simulink library "tpm"  (R2021b)
settings: Solver=VariableStepAuto  StartTime=0.0  StopTime=10.0  RelTol=1e-3
undefined symbols (not defined in the file or in its folder): ENUM_AN_LF, ENUM_AN_LR, ENUM_AN_RF, ENUM_AN_RR, ENUM_POWERSTA_OFF, ENUM_POWERSTA_OFFA, ENUM_POWERSTA_OFFC, ENUM_POWERSTA_ON, ENUM_POWERSTA_READY, ENUM_POWERSTA_STANDBY, ENUM_PWRSTASW_OFF, ENUM_PWRSTASW_OFFA, ENUM_PWRSTASW_OFFCHVCHRG, ENUM_PWRSTASW_STANDBY, ENUM_TPMSSNESORIDREGSTA_START, FALSE, KTPM_DataInVehSpdThreshold_kph, KTPM_Delay_raw8, KTPM_DiagLearn_flg, KTPM_TPMSModelVersion_raw, KTPM_TPMSModelVersionInit_raw, KTPM_WhlRotDir_enum_ovrdflg, KTPM_WhlRotDir_enum_ovrdval, TRUE, ZERO_FLOAT, ZERO_INT
libraries: simulink x58, $bdroot x27, hcu_lib x24
(part 2 of 9)

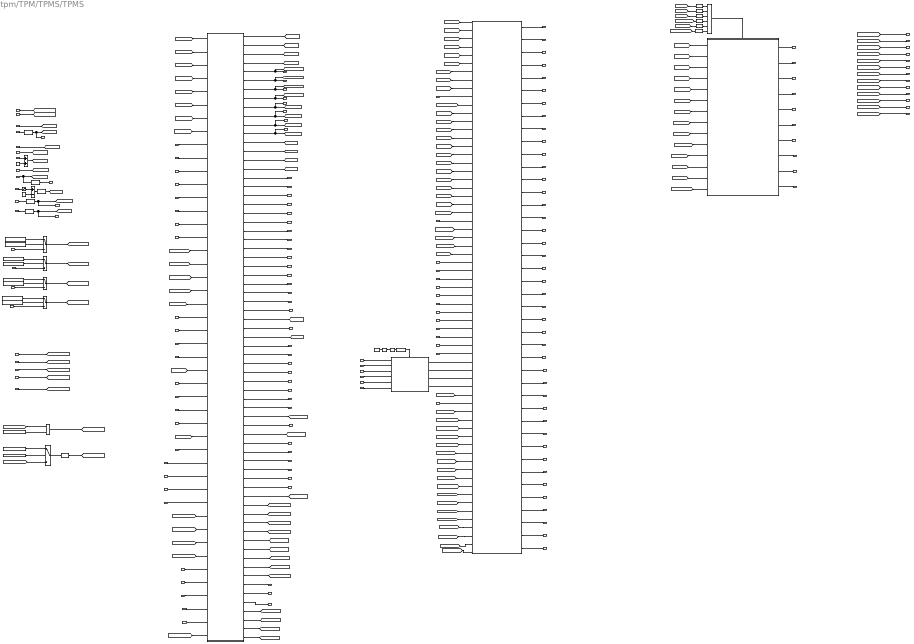
== system tpm/TPM/TPMS/TPMS ==
  note: VINP_RFWhlRotDir_enum
  VPMM_PowerSta_enum : Inport
  VINP_IDin_raw32 : Inport  Port=2
  VINP_DATAin_flg : Inport  Port=3
  VINP_FAT_flg : Inport  Port=4
  VINP_Pin_raw8 : Inport  Port=5
  VINP_Tin_raw8 : Inport  Port=6
  VINP_LFPulseCount_cnt : Inport  Port=7
  VINP_RFPulseCount_cnt : Inport  Port=8
  VINP_LRPulseCount_cnt : Inport  Port=9
  VINP_RRPulseCount_cnt : Inport  Port=10
  VINP_LFPulseCountV_flg : Inport  Port=11
  VINP_RFPulseCountV_flg : Inport  Port=12
  VINP_LRPulseCountV_flg : Inport  Port=13
  VINP_RRPulseCountV_flg : Inport  Port=14
  VINP_BatteryLow_flg : Inport  Port=15
  VTQD_GearActualPosn_enum : Inport  Port=16
  VINP_VehSpeed_kph : Inport  Port=17
  VINP_TPMSResButt_flg : Inport  Port=18
  VINP_TPMSCaliButt_flg : Inport  Port=19
  VINP_IVICANValid_flg : Inport  Port=20
  VINP_TPMSStorge_flg : Inport  Port=21
  VINP_LFID_raw : Inport  Port=22
  VINP_RFID_raw : Inport  Port=23
  VINP_LRID_raw : Inport  Port=24
  VINP_RRID_raw : Inport  Port=25
  VINP_ChkStorge_flg : Inport  Port=26
  VINP_ChkLFID_raw : Inport  Port=27
  VINP_ChkRFID_raw : Inport  Port=28
  VINP_ChkLRID_raw : Inport  Port=29
  VINP_ChkRRID_raw : Inport  Port=30
  VINP_LFWhlRotDir_enum : Inport  Port=31
  VINP_RFWhlRotDir_enum : Inport  Port=32
  VINP_LRWhlRotDir_enum : Inport  Port=33
  VINP_RRWhlRotDir_enum : Inport  Port=34
  VINP_FlashLFSensorFail_flg : Inport  Port=35
  VINP_FlashRFSensorFail_flg : Inport  Port=36
  VINP_FlashLRSensorFail_flg : Inport  Port=37
  VINP_FlashRRSensorFail_flg : Inport  Port=38
  VINP_FlashLFWheelPSW_raw8 : Inport  Port=39
  VINP_FlashRFWheelPSW_raw8 : Inport  Port=40
  VINP_FlashLRWheelPSW_raw8 : Inport  Port=41
  VINP_FlashRRWheelPSW_raw8 : Inport  Port=42
  VINP_FlashLFPindi_enum : Inport  Port=43
  VINP_FlashRFPindi_enum : Inport  Port=44
  VINP_FlashLRPindi_enum : Inport  Port=45
  VINP_FlashRRPindi_enum : Inport  Port=46
  VINP_FlashLFP20_raw8 : Inport  Port=47
  VINP_FlashRFP20_raw8 : Inport  Port=48
  VINP_FlashLRP20_raw8 : Inport  Port=49
  VINP_FlashRRP20_raw8 : Inport  Port=50
  VINP_FlashLFWheelPress_raw8 : Inport  Port=51
  VINP_FlashRFWheelPress_raw8 : Inport  Port=52
  VINP_FlashLRFWheelPress_raw8 : Inport  Port=53
  VINP_FlashRRWheelPress_raw8 : Inport  Port=54
  VINP_FlashLFWheelTemp_C : Inport  Port=55
  VINP_FlashRFWheelTemp_C : Inport  Port=56
  VINP_FlashLRWheelTemp_C : Inport  Port=57
  VINP_FlashRRWheelTemp_C : Inport  Port=58
  VINP_FlashunlearnSfali_flg : Inport  Port=59
  VINP_S1ID_raw : Inport  Port=60
  VINP_S2ID_raw : Inport  Port=61
  VINP_S3ID_raw : Inport  Port=62
  VINP_S4ID_raw : Inport  Port=63
  VINP_Prepresstemptrust_flg : Inport  Port=64
  VINP_TPMSTrigger_flg : Inport  Port=65
  VINP_TPMSSensorIDRegSta_enum : Inport  Port=66
  VINP_FlashTPMModelVersion_raw : Inport  Port=67
  VINP_FlashTPMModelVersionChkSum_raw : Inport  Port=68
  Add : Sum  OutDataTypeStr=int8
  Add1 : Sum  Inputs=+-
  Cast To Boolean : DataTypeConversion  OutDataTypeStr=boolean
  Constant : Constant  Value=-40
  Constant1 : Constant  Value=59
  Constant{5,7,10..11} (4 alike) : Constant  Value=KTPM_WhlRotDir_enum_ovrdflg
  Constant12 : Constant  Value=ENUM_TPMSSNESORIDREGSTA_START
  Constant13 : Constant  Value=TRUE
  Constant{2..4,6} (4 alike) : Constant  Value=KTPM_WhlRotDir_enum_ovrdval
  Constant8 : Constant  Value=KTPM_DiagLearn_flg
  Constant9 : Constant  Value=TRUE
  Data Type Conversion : DataTypeConversion  OutDataTypeStr=uint8
  Data Type Conversion1 : DataTypeConversion  OutDataTypeStr=uint32
  Data Type Conversion2 : DataTypeConversion  OutDataTypeStr=boolean
  Data Type Conversion3 : DataTypeConversion  OutDataTypeStr=boolean
  Data Type Conversion4 : DataTypeConversion  OutDataTypeStr=boolean
  Delay : Delay
  Detect Increase{,1..6} (7 alike) : simulink/Logic and Bit Operations/Detect Increase  vinit=0.0  OutDataTypeStr=boolean
  Equal : RelationalOperator  Operator===  OutDataTypeStr=boolean  RndMeth=Simplest
  GetFlashWheelTemp : Subsystem
  Learn : Subsystem
  Logical Operator : Logic  Operator=OR  Inputs=6  AllPortsSameDT=off  OutDataTypeStr=boolean
  Logical Operator1 : Logic  Operator=NOT  AllPortsSameDT=off  OutDataTypeStr=boolean
  Saturation : Saturate  UpperLimit=255  LowerLimit=59
  Send : Subsystem
  Subsystem : Subsystem
  Switch : Switch  Criteria=u2 > Threshold
  Switch{2..5} (4 alike) : Switch  Criteria=u2 ~= 0
  "VTPM_LFBatWarn_flg " : Outport
  "VTPM_RFBatWarn_flg " : Outport  Port=2
  "VTPM_LRBatWarn_flg " : Outport  Port=3
  "VTPM_RRBatWarn_flg " : Outport  Port=4
  VTPM_LFWheelPress_raw8 : Outport  Port=5
  VTPM_RFWheelPress_raw8 : Outport  Port=6
  VTPM_LRWheelPress_raw8 : Outport  Port=7
  VTPM_RRWheelPress_raw8 : Outport  Port=8
  "VTPM_LFWheelTemp_C " : Outport  Port=9
  "VTPM_RFWheelTemp_C " : Outport  Port=10
  "VTPM_LRWheelTemp_C " : Outport  Port=11
  VTPM_RRWheelTemp_C : Outport  Port=12
  VTPM_LFSensorFail_flg : Outport  Port=13
  VTPM_RFSensorFail_flg : Outport  Port=14
  VTPM_LRSensorFail_flg : Outport  Port=15
  VTPM_RRSensorFail_flg : Outport  Port=16
  VTPM_LFWheelDebug_flg : Outport  Port=17
  VTPM_LRWheelDebug_flg : Outport  Port=18
  VTPM_RFWheelDebug_flg : Outport  Port=19
  VTPM_RRWheelDebug_flg : Outport  Port=20
  VTPM_TPMSResButtAllow_flg : Outport  Port=21
  VTPM_TPMSCaliButtAllow_flg : Outport  Port=22
  VTPM_LFPressIndi_enum : Outport  Port=23
  VTPM_RFPressIndi_enum : Outport  Port=24
  VTPM_LRPressIndi_enum : Outport  Port=25
  VTPM_RRPressIndi_enum : Outport  Port=26
  "VTPM_TPMSWarnIndi_enum " : Outport  Port=27
  VTPM_LFWheelTmpIndi_flg : Outport  Port=28
  VTPM_RFWheelTmpIndi_flg : Outport  Port=29
  VTPM_LRWheelTmpIndi_flg : Outport  Port=30
  VTPM_RRWheelTmpIndi_flg : Outport  Port=31
  VTPM_LFWheelPSW_raw8 : Outport  Port=32
  VTPM_LRWheelPSW_raw8 : Outport  Port=33
  VTPM_RFWheelPSW_raw8 : Outport  Port=34
  VTPM_RRWheelPSW_raw8 : Outport  Port=35
  VTPM_CWheelTips_enum : Outport  Port=36
  VTPM_AutoLTips_enum : Outport  Port=37
  VTPM_LFSensorMode_flg : Outport  Port=38
  VTPM_RFSensorMode_flg : Outport  Port=39
  VTPM_LRSensorMode_flg : Outport  Port=40
  VTPM_RRSensorMode_flg : Outport  Port=41
  VTPM_LFS1_cnt : Outport  Port=42
  VTPM_RFS1_cnt : Outport  Port=43
  VTPM_RRS1_cnt : Outport  Port=44
  VTPM_LRS1_cnt : Outport  Port=45
  VTPM_LFS2_cnt : Outport  Port=46
  VTPM_RFS2_cnt : Outport  Port=47
  VTPM_RRS2_cnt : Outport  Port=48
  VTPM_LRS2_cnt : Outport  Port=49
  VTPM_LFS3_cnt : Outport  Port=50
  VTPM_RFS3_cnt : Outport  Port=51
  VTPM_RRS3_cnt : Outport  Port=52
  VTPM_LRS3_cnt : Outport  Port=53
  VTPM_LFS4_cnt : Outport  Port=54
  VTPM_RFS4_cnt : Outport  Port=55
  VTPM_RRS4_cnt : Outport  Port=56
  VTPM_LRS4_cnt : Outport  Port=57
  VTPM_S1ID_raw32 : Outport  Port=58
  VTPM_S2ID_raw32 : Outport  Port=59
  VTPM_S3ID_raw32 : Outport  Port=60
  VTPM_S4ID_raw32 : Outport  Port=61
  VTPM_S1L_enum : Outport  Port=62
  VTPM_S2L_enum : Outport  Port=63
  VTPM_S3L_enum : Outport  Port=64
  VTPM_S4L_enum : Outport  Port=65
  VTPM_ALFin_flg : Outport  Port=66
  VTPM_IDLOCK_flg : Outport  Port=67
  VTPM_LFP20_raw8 : Outport  Port=68
  VTPM_RFP20_raw8 : Outport  Port=69
  VTPM_LRP20_raw8 : Outport  Port=70
  VTPM_RRP20_raw8 : Outport  Port=71
  VTPM_FAT_flg : Outport  Port=72
  VTPM_IDin_raw32 : Outport  Port=73
  VTPM_S1WheelDebugALTU_pct : Outport  Port=74
  VTPM_S2WheelDebugALTU_pct : Outport  Port=75
  VTPM_S3WheelDebugALTU_pct : Outport  Port=76
  VTPM_S4WheelDebugALTU_pct : Outport  Port=77
  VTPM_ID1messageALTU_raw8 : Outport  Port=78
  VTPM_ID2messageALTU_raw8 : Outport  Port=79
  VTPM_ID3messageALTU_raw8 : Outport  Port=80
  VTPM_ID4messageALTU_raw8 : Outport  Port=81
  VTPM_Chkfin_flg : Outport  Port=82
  VTPM_SetIDLoc_flg : Outport  Port=83
  VTPM_TPMSStorge_flg : Outport  Port=84
  VTPM_ChkStorge_flg : Outport  Port=85
  VTPM_TPMSResButt_flg : Outport  Port=86
  VTPM_LFPindi_enum : Outport  Port=87
  VTPM_RFPind_enum : Outport  Port=88
  VTPM_LRPindi_enum : Outport  Port=89
  VTPM_RRPindi_enum : Outport  Port=90
  VTPM_WriteChkLFID_raw : Outport  Port=91
  VTPM_WriteChkRFID_raw : Outport  Port=92
  VTPM_WriteChkLRID_raw : Outport  Port=93
  VTPM_WriteChkRRID_raw : Outport  Port=94
  VTPM_WriteChkfinLFID_raw : Outport  Port=95
  VTPM_WriteChkfinRFID_raw : Outport  Port=96
  VTPM_WriteChkfinLRID_raw : Outport  Port=97
  VTPM_WriteChkfinRRID_raw : Outport  Port=98
  VTPM_Flashchkdatavalid_enum : Outport  Port=99
  VTPM_Flashdatavalid_enum : Outport  Port=100
  VTPM_unlearnSfali_flg : Outport  Port=101
  VTPM_unlearnSfailvalid_enum : Outport  Port=102
  VTPM_Prepresstempvalid_enum : Outport  Port=103
  VTPM_FlashS1ID_raw : Outport  Port=104
  VTPM_FlashS2ID_raw : Outport  Port=105
  VTPM_FlashS3ID_raw : Outport  Port=106
  VTPM_FlashS4ID_raw : Outport  Port=107
  VTPM_FlashIDvalid_enum : Outport  Port=108
  VTPM_WritingCnt_enum : Outport  Port=109
  VTPM_TPMSTLCmd_flg : Outport  Port=110
  VTPM_LProgress_enum : Outport  Port=111
  VTPM_TPMSSensorIDRegStart_flg : Outport  Port=112
  wires:
  Add/1 -> [VINP_Tin_raw8]
  VINP_Tin_raw8/1 -> Add/1
  Constant/1 -> Add/2
  VINP_TPMSCaliButt_flg/1 -> [VINP_TPMSCaliButt_flg]
  VINP_TPMSResButt_flg/1 -> Data Type Conversion4/1
  VINP_IDin_raw32/1 -> Data Type Conversion1/1, [VINP_IDin_raw32]
  VPMM_PowerSta_enum/1 -> [VPMM_PowerSta_enum]
  Constant1/1 -> Add1/2
  VINP_Pin_raw8/1 -> Saturation/1
  Data Type Conversion/1 -> [VINP_Pin_raw8]
  Saturation/1 -> Add1/1
  Add1/1 -> Data Type Conversion/1
  Data Type Conversion1/1 -> VTPM_IDin_raw32/1
  VINP_VehSpeed_kph/1 -> [VINP_VehSpeed_kph]
  Constant10/1 -> Switch4/2
  Constant7/1 -> Switch3/2
  VINP_LRWhlRotDir_enum/1 -> Switch4/3
  Constant3/1 -> Switch2/1
  Constant5/1 -> Switch2/2
  Constant4/1 -> Switch4/1
  VINP_RFWhlRotDir_enum/1 -> Switch2/3
  Constant2/1 -> Switch3/1
  VINP_LFWhlRotDir_enum/1 -> Switch3/3
  VINP_RRWhlRotDir_enum/1 -> Switch5/3
  Constant11/1 -> Switch5/2
  Constant6/1 -> Switch5/1
  Switch5/1 -> [VTPM_RRWhlRotDir_enum]
  Switch4/1 -> [VTPM_LRWhlRotDir_enum]
  Switch2/1 -> [VTPM_RFWhlRotDir_enum]
  Switch3/1 -> [VTPM_LFWhlRotDir_enum]
  [VTPM_LRWhlRotDir_enum] -> Learn/19(VTPM_LRWhlRotDir_enum)
  [VTPM_RRWhlRotDir_enum] -> Learn/20(VTPM_RRWhlRotDir_enum)
  [VTPM_LFWhlRotDir_enum] -> Learn/17(VTPM_LFWhlRotDir_enum)
  [VTPM_RFWhlRotDir_enum] -> Learn/18(VTPM_RFWhlRotDir_enum)
  [VINP_TPMSStorge_flg] -> Learn/21(VINP_TPMSStorge_flg)
  VINP_LFID_raw/1 -> Learn/22(VINP_LFID_raw)
  VINP_RFID_raw/1 -> Learn/23(VINP_RFID_raw)
  VINP_LRID_raw/1 -> Learn/24(VINP_LRID_raw)
  VINP_RRID_raw/1 -> Learn/25(VINP_RRID_raw)
  VINP_ChkLFID_raw/1 -> Learn/27(VINP_ChkLFID_raw)
  VINP_ChkRFID_raw/1 -> Learn/28(VINP_ChkRFID_raw)
  VINP_ChkLRID_raw/1 -> Learn/29(VINP_ChkLRID_raw)
  VINP_ChkRRID_raw/1 -> Learn/30(VINP_ChkRRID_raw)
  Learn/43(VTPM_ID4messageALTU_raw8) -> VTPM_ID4messageALTU_raw8/1
  Learn/5(VTPM_LFWheelPSW_raw8) -> [VTPM_LFWheelPSW_raw8], VTPM_LFWheelPSW_raw8/1
  Learn/6(VTPM_RFWheelPSW_raw8) -> [VTPM_RFWheelPSW_raw8], VTPM_RFWheelPSW_raw8/1
  Learn/7(VTPM_LRWheelPSW_raw8) -> [VTPM_LRWheelPSW_raw8], VTPM_LRWheelPSW_raw8/1
  Learn/8(VTPM_RRWheelPSW_raw8) -> [VTPM_RRWheelPSW_raw8], VTPM_RRWheelPSW_raw8/1
  Learn/9(VTPM_LFLowPind_enum) -> VTPM_LFPindi_enum/1, [VTPM_LFLowPind_enum]
  Learn/10(VTPM_RFLowPind_enum) -> VTPM_RFPind_enum/1, [VTPM_RFLowPind_enum]
  Learn/11(VTPM_LRLowPind_enum) -> VTPM_LRPindi_enum/1, [VTPM_LRLowPind_enum]
  Learn/12(VTPM_RRLowPind_enum) -> VTPM_RRPindi_enum/1, [VTPM_RRLowPind_enum]
  Learn/1(VTPM_S1ID_raw32) -> [VTPM_S1ID_raw32]
  Learn/2(VTPM_S2ID_raw32) -> [VTPM_S2ID_raw32]
  Learn/3(VTPM_S3ID_raw32) -> [VTPM_S3ID_raw32]
  Learn/4(VTPM_S4ID_raw32) -> [VTPM_S4ID_raw32]
  Learn/17(VTPM_LFS1_cnt) -> VTPM_LFS1_cnt/1
  Learn/18(VTPM_RFS1_cnt) -> VTPM_RFS1_cnt/1
  Learn/19(VTPM_RRS1_cnt) -> VTPM_RRS1_cnt/1
  Learn/20(VTPM_LRS1_cnt) -> VTPM_LRS1_cnt/1
  Learn/21(VTPM_LFS2_cnt) -> VTPM_LFS2_cnt/1
  Learn/22(VTPM_RFS2_cnt) -> VTPM_RFS2_cnt/1
  Learn/23(VTPM_RRS2_cnt) -> VTPM_RRS2_cnt/1
  Learn/24(VTPM_LRS2_cnt) -> VTPM_LRS2_cnt/1
  Learn/25(VTPM_LFS3_cnt) -> VTPM_LFS3_cnt/1
  Learn/26(VTPM_RFS3_cnt) -> VTPM_RFS3_cnt/1
  Learn/27(VTPM_RRS3_cnt) -> VTPM_RRS3_cnt/1
  Learn/28(VTPM_LRS3_cnt) -> VTPM_LRS3_cnt/1
  Learn/29(VTPM_LFS4_cnt) -> VTPM_LFS4_cnt/1
  Learn/30(VTPM_RFS4_cnt) -> VTPM_RFS4_cnt/1
  Learn/31(VTPM_RRS4_cnt) -> VTPM_RRS4_cnt/1
  Learn/32(VTPM_LRS4_cnt) -> VTPM_LRS4_cnt/1
  Learn/39(VTPM_S4WheelDebugALTU_pct) -> VTPM_S4WheelDebugALTU_pct/1
  Learn/40(VTPM_ID1messageALTU_raw8) -> VTPM_ID1messageALTU_raw8/1
  Learn/41(VTPM_ID2messageALTU_raw8) -> VTPM_ID2messageALTU_raw8/1
  Learn/42(VTPM_ID3messageALTU_raw8) -> VTPM_ID3messageALTU_raw8/1
  VTQD_GearActualPosn_enum/1 -> [VTQD_GearActualPosn_enum]
  [VINP_ChkStorge_flg] -> Learn/26(VINP_ChkStorge_flg)
  VINP_TPMSStorge_flg/1 -> Data Type Conversion2/1
  VINP_ChkStorge_flg/1 -> Data Type Conversion3/1
  [VTQD_GearActualPosn_enum] -> Send/11(VTQD_GearActualPosn_enum)
  [VTPM_ALFin_flg] -> Send/26(VTPM_ALFin_flg)
  [VINP_TPMSStorge_flg] -> Send/27(VINP_TPMSStorge_flg)
  [VTPM_IDLOCK_flg] -> Send/28(VTPM_IDLOCK_flg)
  [VINP_VehSpeed_kph] -> Send/12(VINP_VehSpeed_kph)
  [VINP_TPMSResButt_flg] -> Send/13(VINP_TPMSResButt_flg)
  [VINP_TPMSCaliButt_flg] -> Send/14(VINP_TPMSCaliButt_flg)
  [VTPM_S1L_enum] -> Send/15(VTPM_S1L_enum)
  [VTPM_S2L_enum] -> Send/16(VTPM_S2L_enum)
  [VTPM_S3L_enum] -> Send/17(VTPM_S3L_enum)
  [VTPM_S4L_enum] -> Send/18(VTPM_S4L_enum)
  [VTPM_Chkfin_flg] -> Send/19(VTPM_Chkfin_flg)
  [VTPM_LFLowPind_enum] -> Send/20(VTPM_LFLowPind_enum)
  [VTPM_RFLowPind_enum] -> Send/21(VTPM_RFLowPind_enum)
  [VTPM_LRLowPind_enum] -> Send/22(VTPM_LRLowPind_enum)
  [VTPM_RRLowPind_enum] -> Send/23(VTPM_RRLowPind_enum)
  [VINP_FAT_flg] -> Send/24(VINP_FAT_flg)
  [VPMM_PowerSta_enum] -> Send/1(VPMM_PowerSta_enum)
  [VTPM_S1ID_raw32] -> Send/2(VTPM_S1ID_raw32)
  [VTPM_S2ID_raw32] -> Send/3(VTPM_S2ID_raw32)
  [VTPM_S3ID_raw32] -> Send/4(VTPM_S3ID_raw32)
  [VTPM_S4ID_raw32] -> Send/5(VTPM_S4ID_raw32)
  [VINP_IDin_raw32] -> Send/6(VINP_IDin_raw32)
  [VINP_DATAin_flg] -> Send/7(VINP_DATAin_flg)
  [VINP_Pin_raw8] -> Send/8(VINP_Pin_raw8)
  [VINP_Tin_raw8] -> Send/9(VINP_Tin_raw8)
  [VINP_ChkStorge_flg] -> Send/29(VINP_ChkStorge_flg)
  VINP_IVICANValid_flg/1 -> Send/25(VINP_IVICANValid_flg)
  VINP_FlashLFSensorFail_flg/1 -> Send/30(VINP_FlashLFSensorFail_flg)
  VINP_FlashRFSensorFail_flg/1 -> Send/31(VINP_FlashRFSensorFail_flg)
  VINP_FlashLRSensorFail_flg/1 -> Send/32(VINP_FlashLRSensorFail_flg)
  VINP_FlashRRSensorFail_flg/1 -> Send/33(VINP_FlashRRSensorFail_flg)
  VINP_FlashLFP20_raw8/1 -> Send/34(VINP_FlashLFP20_raw8)
  VINP_FlashRFP20_raw8/1 -> Send/35(VINP_FlashRFP20_raw8)
  VINP_FlashLRP20_raw8/1 -> Send/36(VINP_FlashLRP20_raw8)
  VINP_FlashRRP20_raw8/1 -> Send/37(VINP_FlashRRP20_raw8)
  VINP_BatteryLow_flg/1 -> Send/10(VINP_BatteryLow_flg)
  VINP_FlashLFWheelPress_raw8/1 -> Send/38(VINP_FlashLFWheelPress_raw8)
  VINP_FlashRFWheelPress_raw8/1 -> Send/39(VINP_FlashRFWheelPress_raw8)
  VINP_FlashLRFWheelPress_raw8/1 -> Send/40(VINP_FlashLRFWheelPress_raw8)
  VINP_FlashRRWheelPress_raw8/1 -> Send/41(VINP_FlashRRWheelPress_raw8)
  [VTPM_S4L_enum] -> Subsystem/8(VTPM_S4L_enum)
  [VTPM_S3L_enum] -> Subsystem/7(VTPM_S3L_enum)
  [VTPM_S2L_enum] -> Subsystem/6(VTPM_S2L_enum)
  [VTPM_S2ID_raw32] -> Subsystem/2(VTPM_S2ID_raw32)
  [VTPM_S4ID_raw32] -> Subsystem/4(VTPM_S4ID_raw32)
  [VTPM_S3ID_raw32] -> Subsystem/3(VTPM_S3ID_raw32)
  [VINP_TPMSResButt_flg] -> Subsystem/13(VINP_TPMSResButt_flg)
  [VTPM_Chkfin_flg] -> Subsystem/10(VTPM_Chkfin_flg)
  [VTPM_S1L_enum] -> Subsystem/5(VTPM_S1L_enum)
  [VINP_TPMSStorge_flg] -> Subsystem/11(VINP_TPMSStorge_flg)
  [VINP_ChkStorge_flg] -> Subsystem/12(VINP_ChkStorge_flg)
  [VTPM_S1ID_raw32] -> Subsystem/1(VTPM_S1ID_raw32)
  [VTPM_ALFin_flg] -> Subsystem/9(VTPM_ALFin_flg)
  Logical Operator/1 -> Subsystem/Enable
  [VINP_TPMSStorge_flg] -> Detect Increase3/1
  Detect Increase3/1 -> Logical Operator/4
  [VTPM_ALFin_flg] -> Detect Increase/1
  [VINP_ChkStorge_flg] -> Detect Increase1/1
  [VTPM_Chkfin_flg] -> Detect Increase2/1
  Detect Increase/1 -> Logical Operator/1
  Detect Increase1/1 -> Logical Operator/2
  Detect Increase2/1 -> Logical Operator/3
  [VINP_TPMSResButt_flg] -> Detect Increase4/1
  Detect Increase4/1 -> Logical Operator/5
  Subsystem/1(VTPM_WriteChkLFID_raw) -> VTPM_WriteChkLFID_raw/1
  Subsystem/2(VTPM_WriteChkRFID_raw) -> VTPM_WriteChkRFID_raw/1
  Subsystem/3(VTPM_WriteChkLRID_raw) -> VTPM_WriteChkLRID_raw/1
  Subsystem/4(VTPM_WriteChkRRID_raw) -> VTPM_WriteChkRRID_raw/1
  Subsystem/5(VTPM_WriteChkfinLFID_raw) -> VTPM_WriteChkfinLFID_raw/1
  Subsystem/6(VTPM_WriteChkfinRFID_raw) -> VTPM_WriteChkfinRFID_raw/1
  Subsystem/7(VTPM_WriteChkfinLRID_raw) -> VTPM_WriteChkfinLRID_raw/1
  Subsystem/8(VTPM_WriteChkfinRRID_raw) -> VTPM_WriteChkfinRRID_raw/1
  Subsystem/9(VTPM_Flashchkdatavalid_enum) -> VTPM_Flashchkdatavalid_enum/1
  Subsystem/10(VTPM_Flashdatavalid_enum) -> VTPM_Flashdatavalid_enum/1
  [VTPM_unlearnSfali_flg] -> Send/46(VTPM_unlearnSfali_flg)
  [VINP_VehSpeed_kph] -> Learn/31(VINP_VehSpeed_kph)
  VINP_FlashunlearnSfali_flg/1 -> Learn/32(VINP_FlashunlearnSfali_flg)
  VINP_RRPulseCountV_flg/1 -> Learn/16(VINP_RRPulseCountV_flg)
  [VINP_TPMSResButt_flg] -> Learn/1(VINP_TPMSResButt_flg)
  [VINP_IDin_raw32] -> Learn/2(VINP_IDin_raw32)
  [VINP_DATAin_flg] -> Learn/3(VINP_DATAin_flg)
  [VINP_Pin_raw8] -> Learn/4(VINP_Pin_raw8)
  [VINP_Tin_raw8] -> Learn/5(VINP_Tin_raw8)
  [VINP_TPMSCaliButt_flg] -> Learn/6(VINP_TPMSCaliButt_flg)
  [VINP_FAT_flg] -> Learn/7(VINP_FAT_flg)
  [VPMM_PowerSta_enum] -> Learn/8(VPMM_PowerSta_enum)
  VINP_LFPulseCount_cnt/1 -> Learn/9(VINP_LFPulseCount_cnt)
  VINP_RFPulseCount_cnt/1 -> Learn/10(VINP_RFPulseCount_cnt)
  VINP_LRPulseCount_cnt/1 -> Learn/11(VINP_LRPulseCount_cnt)
  VINP_RRPulseCount_cnt/1 -> Learn/12(VINP_RRPulseCount_cnt)
  VINP_LFPulseCountV_flg/1 -> Learn/13(VINP_LFPulseCountV_flg)
  VINP_RFPulseCountV_flg/1 -> Learn/14(VINP_RFPulseCountV_flg)
  VINP_LRPulseCountV_flg/1 -> Learn/15(VINP_LRPulseCountV_flg)
  VINP_DATAin_flg/1 -> [VINP_DATAin_flg]
  VINP_FAT_flg/1 -> [VINP_FAT_flg]
  Data Type Conversion2/1 -> VTPM_TPMSStorge_flg/1, [VINP_TPMSStorge_flg]
  Data Type Conversion3/1 -> VTPM_ChkStorge_flg/1, [VINP_ChkStorge_flg]
  Data Type Conversion4/1 -> VTPM_TPMSResButt_flg/1, [VINP_TPMSResButt_flg]
  VINP_FlashLFPindi_enum/1 -> [VINP_FlashLFPindi_enum]
  VINP_FlashRFPindi_enum/1 -> [VINP_FlashRFPindi_enum]
  VINP_FlashLRPindi_enum/1 -> [VINP_FlashLRPindi_enum]
  VINP_FlashRRPindi_enum/1 -> [VINP_FlashRRPindi_enum]
  VINP_FlashLFWheelPSW_raw8/1 -> Learn/33(VINP_FlashLFWheelPSW_raw8)
  VINP_FlashRFWheelPSW_raw8/1 -> Learn/34(VINP_FlashRFWheelPSW_raw8)
  VINP_FlashLRWheelPSW_raw8/1 -> Learn/35(VINP_FlashLRWheelPSW_raw8)
  VINP_FlashRRWheelPSW_raw8/1 -> Learn/36(VINP_FlashRRWheelPSW_raw8)
  [VINP_FlashLFPindi_enum] -> Learn/37(VINP_FlashLFPindi_enum)
  [VINP_FlashRFPindi_enum] -> Learn/38(VINP_FlashRFPindi_enum)
  [VINP_FlashLRPindi_enum] -> Learn/39(VINP_FlashLRPindi_enum)
  [VINP_FlashRRPindi_enum] -> Learn/40(VINP_FlashRRPindi_enum)
  VINP_S3ID_raw/1 -> Learn/43(VINP_S3ID_raw)
  VINP_S4ID_raw/1 -> Learn/44(VINP_S4ID_raw)
  VINP_S2ID_raw/1 -> Learn/42(VINP_S2ID_raw)
  VINP_S1ID_raw/1 -> Learn/41(VINP_S1ID_raw)
  Learn/13(VTPM_S1L_enum) -> [VTPM_S1L_enum]
  Learn/16(VTPM_S4L_enum) -> [VTPM_S4L_enum]
  Learn/14(VTPM_S2L_enum) -> [VTPM_S2L_enum]
  Learn/15(VTPM_S3L_enum) -> [VTPM_S3L_enum]
  Learn/38(VTPM_S3WheelDebugALTU_pct) -> VTPM_S3WheelDebugALTU_pct/1
  Learn/33(VTPM_IDLOCK_flg) -> [VTPM_IDLOCK_flg]
  Learn/34(VTPM_FATAND_flg) -> VTPM_FAT_flg/1
  Learn/35(VTPM_ALFin_flg) -> [VTPM_ALFin_flg]
  Learn/36(VTPM_S1WheelDebugALTU_pct) -> VTPM_S1WheelDebugALTU_pct/1
  Learn/37(VTPM_S2WheelDebugALTU_pct) -> VTPM_S2WheelDebugALTU_pct/1
  Learn/44(VTPM_Chkfin_flg) -> [VTPM_Chkfin_flg]
  Learn/45(VTPM_SetIDLoc_flg) -> VTPM_SetIDLoc_flg/1
  Learn/46(VTPM_unlearnSfali_flg) -> [VTPM_unlearnSfali_flg]
  Learn/47(VTPM_unlearnSfailvalid_enum) -> VTPM_unlearnSfailvalid_enum/1
  Learn/48(VTPM_FlashS1ID_raw) -> VTPM_FlashS1ID_raw/1
  Learn/49(VTPM_FlashS2ID_raw) -> VTPM_FlashS2ID_raw/1
  Learn/50(VTPM_FlashS3ID_raw) -> VTPM_FlashS3ID_raw/1
  Learn/51(VTPM_FlashS4ID_raw) -> VTPM_FlashS4ID_raw/1
  Learn/52(VTPM_FlashIDvalid_enum) -> VTPM_FlashIDvalid_enum/1
  [VTPM_S1ID_raw32] -> VTPM_S1ID_raw32/1
  [VTPM_S2ID_raw32] -> VTPM_S2ID_raw32/1
  [VTPM_S3ID_raw32] -> VTPM_S3ID_raw32/1
  [VTPM_S4ID_raw32] -> VTPM_S4ID_raw32/1
  [VTPM_S1L_enum] -> VTPM_S1L_enum/1
  [VTPM_S2L_enum] -> VTPM_S2L_enum/1
  [VTPM_S3L_enum] -> VTPM_S3L_enum/1
  [VTPM_S4L_enum] -> VTPM_S4L_enum/1
  [VTPM_ALFin_flg] -> VTPM_ALFin_flg/1
  [VTPM_IDLOCK_flg] -> VTPM_IDLOCK_flg/1
  [VTPM_unlearnSfali_flg] -> VTPM_unlearnSfali_flg/1
  [VTPM_Chkfin_flg] -> VTPM_Chkfin_flg/1
  VINP_Prepresstemptrust_flg/1 -> Send/47(VINP_Prepresstemptrust_flg)
  Learn/53(VTPM_unlockpopup_flg) -> [VTPM_unlockpopup_flg]
  [VTPM_unlockpopup_flg] -> Send/48(VTPM_unlockpopup_flg)
  Learn/63(VTPM_WritingCnt_enum) -> VTPM_WritingCnt_enum/1
  Learn/64(VTPM_TPMSTLCmd_flg) -> VTPM_TPMSTLCmd_flg/1
  Learn/62(VTPM_TPMSmanualDone_flg) -> [VTPM_TPMSmanualDone_flg]
  Learn/61(VTPM_ManualID4Temp_C) -> [VTPM_ManualID4Temp_C]
  Learn/65(VTPM_LProgress_enum) -> VTPM_LProgress_enum/1
  Learn/60(VTPM_ManualID3Temp_C) -> [VTPM_ManualID3Temp_C]
  Learn/59(VTPM_ManualID2Temp_C) -> [VTPM_ManualID2Temp_C]
  Learn/58(VTPM_ManualID1Temp_C) -> [VTPM_ManualID1Temp_C]
  Learn/57(VTPM_ManualID4pressure_raw) -> [VTPM_ManualID4pressure_raw]
  Learn/54(VTPM_ManualID1pressure_raw) -> [VTPM_ManualID1pressure_raw]
  Learn/55(VTPM_ManualID2pressure_raw) -> [VTPM_ManualID2pressure_raw]
  Learn/56(VTPM_ManualID3pressure_raw) -> [VTPM_ManualID3pressure_raw]
  [VTPM_ManualID4Temp_C] -> Send/56(VTPM_ManualID4Temp_C)
  [VTPM_ManualID1Temp_C] -> Send/53(VTPM_ManualID1Temp_C)
  [VTPM_ManualID3Temp_C] -> Send/55(VTPM_ManualID3Temp_C)
  [VTPM_ManualID2Temp_C] -> Send/54(VTPM_ManualID2Temp_C)
  [VTPM_ManualID1pressure_raw] -> Send/49(VTPM_ManualID1pressure_raw)
  [VTPM_ManualID2pressure_raw] -> Send/50(VTPM_ManualID2pressure_raw)
  [VTPM_ManualID3pressure_raw] -> Send/51(VTPM_ManualID3pressure_raw)
  [VTPM_ManualID4pressure_raw] -> Send/52(VTPM_ManualID4pressure_raw)
  [VTPM_TPMSmanualDone_flg] -> Send/57(VTPM_TPMSmanualDone_flg)
  Send/1("VTPM_LFBatWarn_flg ") -> "VTPM_LFBatWarn_flg "/1
  Send/2("VTPM_RFBatWarn_flg ") -> "VTPM_RFBatWarn_flg "/1
  Send/3("VTPM_LRBatWarn_flg ") -> "VTPM_LRBatWarn_flg "/1
  Send/4(VTPM_RRBatWarn_flg) -> "VTPM_RRBatWarn_flg "/1
  Send/5(VTPM_LFWheelPress_raw8) -> VTPM_LFWheelPress_raw8/1
  Send/6(VTPM_RFWheelPress_raw8) -> VTPM_RFWheelPress_raw8/1
  Send/7(VTPM_LRWheelPress_raw8) -> VTPM_LRWheelPress_raw8/1
  Send/8(VTPM_RRWheelPress_raw8) -> VTPM_RRWheelPress_raw8/1
  Send/9(VTPM_LFWheelTemp_C) -> "VTPM_LFWheelTemp_C "/1
  Send/10(VTPM_RFWheelTemp_C) -> "VTPM_RFWheelTemp_C "/1
  Send/11(VTPM_LRWheelTemp_C) -> "VTPM_LRWheelTemp_C "/1
  Send/12(VTPM_RRWheelTemp_C) -> VTPM_RRWheelTemp_C/1
  Send/13(VTPM_LFSensorFail_flg) -> VTPM_LFSensorFail_flg/1
  Send/14(VTPM_RFSensorFail_flg) -> VTPM_RFSensorFail_flg/1
  Send/15(VTPM_LRSensorFail_flg) -> VTPM_LRSensorFail_flg/1
  Send/16(VTPM_RRSensorFail_flg) -> VTPM_RRSensorFail_flg/1
  Send/17(VTPM_LFWheelDebug_flg) -> VTPM_LFWheelDebug_flg/1
  Send/18(VTPM_LRWheelDebug_flg) -> VTPM_LRWheelDebug_flg/1
  Send/19(VTPM_RFWheelDebug_flg) -> VTPM_RFWheelDebug_flg/1
  Send/20(VTPM_RRWheelDebug_flg) -> VTPM_RRWheelDebug_flg/1
  Send/21(VTPM_TPMSResButtAllow_flg) -> VTPM_TPMSResButtAllow_flg/1
  Send/22(VTPM_TPMSCaliButtAllow_flg) -> VTPM_TPMSCaliButtAllow_flg/1
  Send/23(VTPM_LFPressIndi_enum) -> VTPM_LFPressIndi_enum/1
  Send/24(VTPM_RFPressIndi_enum) -> VTPM_RFPressIndi_enum/1
  Send/25(VTPM_LRPressIndi_enum) -> VTPM_LRPressIndi_enum/1
  Send/26(VTPM_RRPressIndi_enum) -> VTPM_RRPressIndi_enum/1
  Send/27("VTPM_TPMSWarnIndi_enum ") -> "VTPM_TPMSWarnIndi_enum "/1
  Send/28(VTPM_LFWheelTmpIndi_flg) -> VTPM_LFWheelTmpIndi_flg/1
  Send/29(VTPM_RFWheelTmpIndi_flg) -> VTPM_RFWheelTmpIndi_flg/1
  Send/30(VTPM_LRWheelTmpIndi_flg) -> VTPM_LRWheelTmpIndi_flg/1
  Send/31(VTPM_RRWheelTmpIndi_flg) -> VTPM_RRWheelTmpIndi_flg/1
  Send/32(VTPM_CWheelTips_enum) -> VTPM_CWheelTips_enum/1
  Send/33(VTPM_AutoLTips_enum) -> VTPM_AutoLTips_enum/1
  Send/34(VTPM_LFSensorMode_flg) -> VTPM_LFSensorMode_flg/1
  Send/35(VTPM_RFSensorMode_flg) -> VTPM_RFSensorMode_flg/1
  Send/36(VTPM_LRSensorMode_flg) -> VTPM_LRSensorMode_flg/1
  Send/37(VTPM_RRSensorMode_flg) -> VTPM_RRSensorMode_flg/1
  Send/38(VTPM_LFP20_raw8) -> VTPM_LFP20_raw8/1
  Send/39(VTPM_RFP20_raw8) -> VTPM_RFP20_raw8/1
  Send/40(VTPM_LRP20_raw8) -> VTPM_LRP20_raw8/1
  Send/41(VTPM_RRP20_raw8) -> VTPM_RRP20_raw8/1
  Send/42(VTPM_Prepresstempvalid_enum) -> VTPM_Prepresstempvalid_enum/1
  [VTPM_TPMSmanualDone_flg] -> Subsystem/14(VTPM_TPMSmanualDone_flg)
  Detect Increase5/1 -> Logical Operator/6
  [VTPM_TPMSmanualDone_flg] -> Detect Increase5/1
  VINP_TPMSTrigger_flg/1 -> Learn/45(VINP_TPMSTrigger_flg)
  Constant9/1 -> Switch/1
  Constant8/1 -> Switch/2
  VINP_TPMSSensorIDRegSta_enum/1 -> [VINP_TPMSSensorIDRegSta_enum]
  [VTPM_DiagLearn_flg] -> Learn/46(VTPM_DiagLearn_flg)
  [VINP_TPMSSensorIDRegSta_enum] -> Equal/1
  Constant12/1 -> Equal/2
  Detect Increase6/1 -> [VTPM_DiagLearn_flg]
  Switch/1 -> Detect Increase6/1
  [VTPM_TPMSSensorIDRegStart_flg] -> VTPM_TPMSSensorIDRegStart_flg/1
  Equal/1 -> [VTPM_TPMSSensorIDRegStart_flg]  "VTPM_TPMSSensorIDRegStart_flg"
  [VTPM_TPMSSensorIDRegStart_flg] -> Switch/3
  [VTPM_LFWheelPSW_raw8] -> Send/58(VTPM_LFWheelPSW_raw8)
  [VTPM_RFWheelPSW_raw8] -> Send/59(VTPM_RFWheelPSW_raw8)
  [VTPM_LRWheelPSW_raw8] -> Send/60(VTPM_LRWheelPSW_raw8)
  [VTPM_RRWheelPSW_raw8] -> Send/61(VTPM_RRWheelPSW_raw8)
  Learn/66(VTPM_ManualLFP20_raw8) -> [VTPM_ManualLFP20_raw8]
  Learn/67(VTPM_ManualRFP20_raw8) -> [VTPM_ManualRFP20_raw8]
  Learn/68(VTPM_ManualLRP20_raw8) -> [VTPM_ManualLRP20_raw8]
  Learn/69(VTPM_ManualRRP20_raw8) -> [VTPM_ManualRRP20_raw8]
  [VTPM_ManualLFP20_raw8] -> Send/62(VTPM_ManualLFP20_raw8)
  [VTPM_ManualRFP20_raw8] -> Send/63(VTPM_ManualRFP20_raw8)
  [VTPM_ManualLRP20_raw8] -> Send/64(VTPM_ManualLRP20_raw8)
  [VTPM_ManualRRP20_raw8] -> Send/65(VTPM_ManualRRP20_raw8)
  VINP_FlashLFWheelTemp_C/1 -> GetFlashWheelTemp/1(VINP_FlashLFWheelTemp_C)
  VINP_FlashRFWheelTemp_C/1 -> GetFlashWheelTemp/2(VINP_FlashRFWheelTemp_C)
  VINP_FlashLRWheelTemp_C/1 -> GetFlashWheelTemp/3(VINP_FlashLRWheelTemp_C)
  VINP_FlashRRWheelTemp_C/1 -> GetFlashWheelTemp/4(VINP_FlashRRWheelTemp_C)
  GetFlashWheelTemp/1(VTPM_HandledFlashLFWTemp_C) -> Send/42(VINP_FlashLFWheelTemp_C)
  GetFlashWheelTemp/2(VTPM_HandledFlashRFWTemp_C) -> Send/43(VINP_FlashRFWheelTemp_C)
  GetFlashWheelTemp/3(VTPM_HandledFlashLRWTemp_C) -> Send/44(VINP_FlashLRWheelTemp_C)
  GetFlashWheelTemp/4(VTPM_HandledFlashRRWTemp_C) -> Send/45(VINP_FlashRRWheelTemp_C)
  VINP_FlashTPMModelVersion_raw/1 -> GetFlashWheelTemp/5(VINP_FlashTPMModelVersion_raw)
  VINP_FlashTPMModelVersionChkSum_raw/1 -> GetFlashWheelTemp/6(VINP_FlashTPMModelVersionChkSum_raw)
  Constant13/1 -> Delay/1
  Cast To Boolean/1 -> GetFlashWheelTemp/Enable
  Logical Operator1/1 -> Cast To Boolean/1
  Delay/1 -> Logical Operator1/1

== system tpm/TPM/TPMS/ModelVersion/Subsystem ==
  KTPM_TPMSModelVersion_raw : Inport
  Enable : EnablePort
  Add : Sum  Inputs=+++
  Add1 : Sum  Inputs=+-
  Add3 : Sum  Inputs=+--
  Cast To Single : DataTypeConversion  OutDataTypeStr=single
  Cast To Single1 : DataTypeConversion  OutDataTypeStr=single
  Cast To Single2 : DataTypeConversion  OutDataTypeStr=single
  Constant : Constant  Value=1000
  Constant1 : Constant  Value=3
  Constant2 : Constant  Value=5
  Constant3 : Constant  Value=7
  Data Type Conversion{,1..3} (4 alike) : DataTypeConversion  OutDataTypeStr=uint8
  Gain : Gain  Gain=0.01
  Gain1 : Gain  Gain=10
  Gain2 : Gain  Gain=0.1
  Gain3 : Gain  Gain=100
  Gain4 : Gain  Gain=10
  ModMath : hcu_lib/Basic_Blocks/ModMath
  Product : Product
  Product1 : Product
  Product2 : Product
  VTPM_ModelVersion_raw : Outport
  VTPM_ModelVersionChksum_raw : Outport  Port=2
  wires:
  Gain4/1 -> Add3/3
  [VTPM_VersionHundreds_raw] -> Product/1
  [VTPM_VersionHundreds_raw] -> Gain1/1
  Constant1/1 -> Product/2
  [VTPM_VersionHundreds_raw] -> Gain3/1
  [VTPM_VersionTens_raw] -> Gain4/1
  KTPM_TPMSModelVersion_raw/1 -> VTPM_ModelVersion_raw/1, Cast To Single/1
  [VTPM_VersionTens_raw] -> Product1/1
  Data Type Conversion/1 -> [VTPM_VersionHundreds_raw]
  Gain2/1 -> Add1/1
  Constant3/1 -> Product2/2
  Product1/1 -> Add/2
  [VTPM_VersionUnits_raw] -> Product2/1
  Product2/1 -> Add/3
  Constant2/1 -> Product1/2
  ModMath/1 -> Data Type Conversion2/1
  Product/1 -> Add/1
  Constant/1 -> Cast To Single2/1
  Add/1 -> Cast To Single1/1
  Data Type Conversion1/1 -> [VTPM_VersionTens_raw]
  Data Type Conversion3/1 -> [VTPM_VersionUnits_raw]
  Gain1/1 -> Add1/2
  Add3/1 -> Data Type Conversion3/1
  Add1/1 -> Data Type Conversion1/1
  Gain/1 -> Data Type Conversion/1
  Gain3/1 -> Add3/2
  Data Type Conversion2/1 -> VTPM_ModelVersionChksum_raw/1
  Cast To Single/1 -> Add3/1, Gain2/1, Gain/1
  Cast To Single1/1 -> ModMath/1
  Cast To Single2/1 -> ModMath/2

== system tpm/TPM/TPMS/TPMS/GetFlashWheelTemp ==
  VINP_FlashLFWheelTemp_C : Inport
  VINP_FlashRFWheelTemp_C : Inport  Port=2
  VINP_FlashLRWheelTemp_C : Inport  Port=3
  VINP_FlashRRWheelTemp_C : Inport  Port=4
  VINP_FlashTPMModelVersion_raw : Inport  Port=5
  VINP_FlashTPMModelVersionChkSum_raw : Inport  Port=6
  Enable : EnablePort
  Add : Sum  Inputs=+++
  Add{1..3,7} (4 alike) : Sum
  Add5 : Sum  Inputs=+-
  Add6 : Sum  Inputs=+--
  Cast To Single{,1..10} (11 alike) : DataTypeConversion  OutDataTypeStr=single
  Constant : Constant  Value=3
  Constant1 : Constant  Value=5
  Constant{9..11,13} (4 alike) : Constant  Value=-40
  Constant2 : Constant  Value=7
  Constant3 : Constant  Value=KTPM_TPMSModelVersionInit_raw
  Constant8 : Constant  Value=1000  OutDataTypeStr=uint16
  Data Type Conversion{,1..3} (4 alike) : DataTypeConversion  OutDataTypeStr=uint8
  Equal : RelationalOperator  Operator===  OutDataTypeStr=boolean  RndMeth=Simplest
  Equal1 : RelationalOperator  OutDataTypeStr=boolean  RndMeth=Simplest
  Gain : Gain  Gain=0.01
  Gain1 : Gain  Gain=10
  Gain2 : Gain  Gain=0.1
  Gain3 : Gain  Gain=100
  Gain4 : Gain  Gain=10
  Logical Operator : Logic  AllPortsSameDT=off  OutDataTypeStr=boolean
  ModMath : hcu_lib/Basic_Blocks/ModMath
  Product : Product
  Product1 : Product
  Product2 : Product
  Switch{,1..3} (4 alike) : Switch  Criteria=u2 > Threshold
  VTPM_HandledFlashLFWTemp_C : Outport
  VTPM_HandledFlashRFWTemp_C : Outport  Port=2
  VTPM_HandledFlashLRWTemp_C : Outport  Port=3
  VTPM_HandledFlashRRWTemp_C : Outport  Port=4
  wires:
  VINP_FlashLFWheelTemp_C/1 -> Cast To Single2/1
  Constant13/1 -> Add7/2
  VINP_FlashTPMModelVersionChkSum_raw/1 -> Equal/2
  Equal/1 -> Logical Operator/2
  [VTPM_FlashModelVersionValid] -> Switch/2
  Add7/1 -> Cast To Single7/1
  Switch/1 -> VTPM_HandledFlashLFWTemp_C/1
  Switch1/1 -> VTPM_HandledFlashRFWTemp_C/1
  VINP_FlashRFWheelTemp_C/1 -> Cast To Single/1
  [VTPM_FlashModelVersionValid] -> Switch1/2
  Constant9/1 -> Add2/2
  Add2/1 -> Cast To Single8/1
  VINP_FlashLRWheelTemp_C/1 -> Cast To Single1/1
  Constant10/1 -> Add1/2
  Add1/1 -> Cast To Single9/1
  [VTPM_FlashModelVersionValid] -> Switch2/2
  Switch2/1 -> VTPM_HandledFlashLRWTemp_C/1
  VINP_FlashRRWheelTemp_C/1 -> Cast To Single3/1
  Switch3/1 -> VTPM_HandledFlashRRWTemp_C/1
  Add3/1 -> Cast To Single10/1
  [VTPM_FlashModelVersionValid] -> Switch3/2
  Constant11/1 -> Add3/2
  VINP_FlashTPMModelVersion_raw/1 -> [VINP_FlashTPMModelVersion_raw], Cast To Single4/1
  Add5/1 -> Data Type Conversion1/1
  Gain/1 -> Data Type Conversion/1
  Gain3/1 -> Add6/2
  Add/1 -> Cast To Single5/1
  Add6/1 -> Data Type Conversion3/1
  Gain1/1 -> Add5/2
  Constant8/1 -> Cast To Single6/1
  Data Type Conversion3/1 -> [VTPM_VersionUnits_raw]
  Product/1 -> Add/1
  [VTPM_VersionUnits_raw] -> Product2/1
  Product1/1 -> Add/2
  Constant2/1 -> Product2/2
  Constant1/1 -> Product1/2
  Product2/1 -> Add/3
  ModMath/1 -> Data Type Conversion2/1
  Data Type Conversion1/1 -> [VTPM_VersionTens_raw]
  Data Type Conversion/1 -> [VTPM_VersionHundreds_raw]
  Gain2/1 -> Add5/1
  [VTPM_VersionTens_raw] -> Product1/1
  [VTPM_VersionHundreds_raw] -> Gain3/1
  Constant/1 -> Product/2
  [VTPM_VersionHundreds_raw] -> Product/1
  Data Type Conversion2/1 -> Equal/1
  Gain4/1 -> Add6/3
  [VTPM_VersionHundreds_raw] -> Gain1/1
  [VTPM_VersionTens_raw] -> Gain4/1
  Cast To Single2/1 -> Add7/1, Switch/3
  Cast To Single/1 -> Add2/1, Switch1/3
  Cast To Single1/1 -> Add1/1, Switch2/3
  Cast To Single3/1 -> Add3/1, Switch3/3
  Cast To Single4/1 -> Add6/1, Gain2/1, Gain/1
  Cast To Single5/1 -> ModMath/1
  Cast To Single6/1 -> ModMath/2
  Cast To Single7/1 -> Switch/1
  Cast To Single8/1 -> Switch1/1
  Cast To Single9/1 -> Switch2/1
  Cast To Single10/1 -> Switch3/1
  [VINP_FlashTPMModelVersion_raw] -> Equal1/1
  Equal1/1 -> Logical Operator/1
  Constant3/1 -> Equal1/2
  Logical Operator/1 -> [VTPM_FlashModelVersionValid]

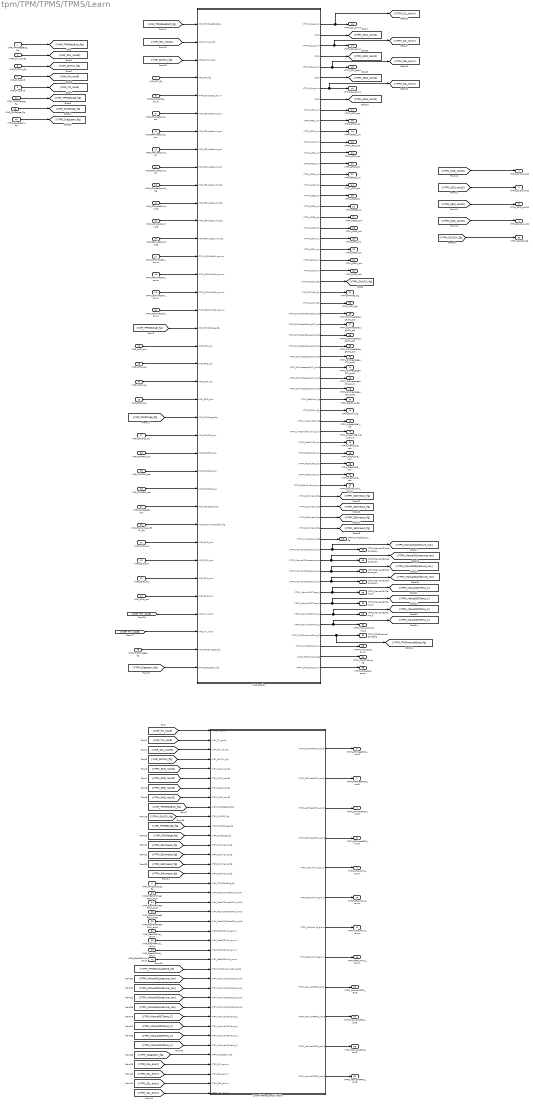
== system tpm/TPM/TPMS/TPMS/Learn ==
  VINP_TPMSResButt_flg : Inport
  VINP_IDin_raw32 : Inport  Port=2
  VINP_DATAin_flg : Inport  Port=3
  VINP_Pin_raw8 : Inport  Port=4
  VINP_Tin_raw8 : Inport  Port=5
  VINP_TPMSCaliButt_flg : Inport  Port=6
  VINP_FAT_flg : Inport  Port=7
  VPMM_PowerSta_enum : Inport  Port=8
  VINP_LFPulseCount_cnt : Inport  Port=9
  VINP_RFPulseCount_cnt : Inport  Port=10
  VINP_LRPulseCount_cnt : Inport  Port=11
  VINP_RRPulseCount_cnt : Inport  Port=12
  VINP_LFPulseCountV_flg : Inport  Port=13
  VINP_RFPulseCountV_flg : Inport  Port=14
  VINP_LRPulseCountV_flg : Inport  Port=15
  VINP_RRPulseCountV_flg : Inport  Port=16
  VTPM_LFWhlRotDir_enum : Inport  Port=17
  VTPM_RFWhlRotDir_enum : Inport  Port=18
  VTPM_LRWhlRotDir_enum : Inport  Port=19
  VTPM_RRWhlRotDir_enum : Inport  Port=20
  VINP_TPMSStorge_flg : Inport  Port=21
  VINP_LFID_raw : Inport  Port=22
  VINP_RFID_raw : Inport  Port=23
  VINP_LRID_raw : Inport  Port=24
  VINP_RRID_raw : Inport  Port=25
  VINP_ChkStorge_flg : Inport  Port=26
  VINP_ChkLFID_raw : Inport  Port=27
  VINP_ChkRFID_raw : Inport  Port=28
  VINP_ChkLRID_raw : Inport  Port=29
  VINP_ChkRRID_raw : Inport  Port=30
  VINP_VehSpeed_kph : Inport  Port=31
  VINP_FlashunlearnSfali_flg : Inport  Port=32
  VINP_FlashLFWheelPSW_raw8 : Inport  Port=33
  VINP_FlashRFWheelPSW_raw8 : Inport  Port=34
  VINP_FlashLRWheelPSW_raw8 : Inport  Port=35
  VINP_FlashRRWheelPSW_raw8 : Inport  Port=36
  VINP_FlashLFPindi_enum : Inport  Port=37
  VINP_FlashRFPindi_enum : Inport  Port=38
  VINP_FlashLRPindi_enum : Inport  Port=39
  VINP_FlashRRPindi_enum : Inport  Port=40
  VINP_S1ID_raw : Inport  Port=41
  VINP_S2ID_raw : Inport  Port=42
  VINP_S3ID_raw : Inport  Port=43
  VINP_S4ID_raw : Inport  Port=44
  VINP_TPMSTrigger_flg : Inport  Port=45
  VTPM_DiagLearn_flg : Inport  Port=46
  AutoLocation : Subsystem
  LowerTirePressureCalibration : Subsystem
  VTPM_S1ID_raw32 : Outport
  VTPM_S2ID_raw32 : Outport  Port=2
  VTPM_S3ID_raw32 : Outport  Port=3
  VTPM_S4ID_raw32 : Outport  Port=4
  VTPM_LFWheelPSW_raw8 : Outport  Port=5
  VTPM_RFWheelPSW_raw8 : Outport  Port=6
  VTPM_LRWheelPSW_raw8 : Outport  Port=7
  VTPM_RRWheelPSW_raw8 : Outport  Port=8
  VTPM_LFLowPind_enum : Outport  Port=9
  VTPM_RFLowPind_enum : Outport  Port=10
  VTPM_LRLowPind_enum : Outport  Port=11
  VTPM_RRLowPind_enum : Outport  Port=12
  VTPM_S1L_enum : Outport  Port=13
  VTPM_S2L_enum : Outport  Port=14
  VTPM_S3L_enum : Outport  Port=15
  VTPM_S4L_enum : Outport  Port=16
  VTPM_LFS1_cnt : Outport  Port=17
  VTPM_RFS1_cnt : Outport  Port=18
  VTPM_RRS1_cnt : Outport  Port=19
  VTPM_LRS1_cnt : Outport  Port=20
  VTPM_LFS2_cnt : Outport  Port=21
  VTPM_RFS2_cnt : Outport  Port=22
  VTPM_RRS2_cnt : Outport  Port=23
  VTPM_LRS2_cnt : Outport  Port=24
  VTPM_LFS3_cnt : Outport  Port=25
  VTPM_RFS3_cnt : Outport  Port=26
  VTPM_RRS3_cnt : Outport  Port=27
  VTPM_LRS3_cnt : Outport  Port=28
  VTPM_LFS4_cnt : Outport  Port=29
  VTPM_RFS4_cnt : Outport  Port=30
  VTPM_RRS4_cnt : Outport  Port=31
  VTPM_LRS4_cnt : Outport  Port=32
  VTPM_IDLOCK_flg : Outport  Port=33
  VTPM_FATAND_flg : Outport  Port=34
  VTPM_ALFin_flg : Outport  Port=35
  VTPM_S1WheelDebugALTU_pct : Outport  Port=36
  VTPM_S2WheelDebugALTU_pct : Outport  Port=37
  VTPM_S3WheelDebugALTU_pct : Outport  Port=38
  VTPM_S4WheelDebugALTU_pct : Outport  Port=39
  VTPM_ID1messageALTU_raw8 : Outport  Port=40
  VTPM_ID2messageALTU_raw8 : Outport  Port=41
  VTPM_ID3messageALTU_raw8 : Outport  Port=42
  VTPM_ID4messageALTU_raw8 : Outport  Port=43
  VTPM_Chkfin_flg : Outport  Port=44
  VTPM_SetIDLoc_flg : Outport  Port=45
  VTPM_unlearnSfali_flg : Outport  Port=46
  VTPM_unlearnSfailvalid_enum : Outport  Port=47
  VTPM_FlashS1ID_raw : Outport  Port=48
  VTPM_FlashS2ID_raw : Outport  Port=49
  VTPM_FlashS3ID_raw : Outport  Port=50
  VTPM_FlashS4ID_raw : Outport  Port=51
  VTPM_FlashIDvalid_enum : Outport  Port=52
  VTPM_unlockpopup_flg : Outport  Port=53
  VTPM_ManualID1pressure_raw : Outport  Port=54
  VTPM_ManualID2pressure_raw : Outport  Port=55
  VTPM_ManualID3pressure_raw : Outport  Port=56
  VTPM_ManualID4pressure_raw : Outport  Port=57
  VTPM_ManualID1Temp_C : Outport  Port=58
  VTPM_ManualID2Temp_C : Outport  Port=59
  VTPM_ManualID3Temp_C : Outport  Port=60
  VTPM_ManualID4Temp_C : Outport  Port=61
  VTPM_TPMSmanualDone_flg : Outport  Port=62
  VTPM_WritingCnt_enum : Outport  Port=63
  VTPM_TPMSTLCmd_flg : Outport  Port=64
  VTPM_LProgress_enum : Outport  Port=65
  VTPM_ManualLFP20_raw8 : Outport  Port=66
  VTPM_ManualRFP20_raw8 : Outport  Port=67
  VTPM_ManualLRP20_raw8 : Outport  Port=68
  VTPM_ManualRRP20_raw8 : Outport  Port=69
  wires:
  VINP_IDin_raw32/1 -> [VINP_IDin_raw32]
  VINP_DATAin_flg/1 -> [VINP_DATAin_flg]
  VINP_TPMSResButt_flg/1 -> [VINP_TPMSResButt_flg]
  [VTPM_S1ID_raw32] -> VTPM_S1ID_raw32/1
  [VTPM_S2ID_raw32] -> VTPM_S2ID_raw32/1
  [VTPM_S3ID_raw32] -> VTPM_S3ID_raw32/1
  [VTPM_S4ID_raw32] -> VTPM_S4ID_raw32/1
  VINP_Pin_raw8/1 -> [VINP_Pin_raw8]
  VINP_Tin_raw8/1 -> [VINP_Tin_raw8]
  VINP_ChkStorge_flg/1 -> [VINP_ChkStorge_flg]
  VINP_TPMSStorge_flg/1 -> [VINP_TPMSStorge_flg]
  [VINP_Pin_raw8] -> LowerTirePressureCalibration/1(VINP_Pin_raw8)
  [VINP_Tin_raw8] -> LowerTirePressureCalibration/2(VINP_Tin_raw8)
  [VINP_IDin_raw32] -> LowerTirePressureCalibration/3(VINP_IDin_raw32)
  [VTPM_S1ID_raw32] -> LowerTirePressureCalibration/5(VTPM_S1ID_raw32)
  [VINP_DATAin_flg] -> LowerTirePressureCalibration/4(VINP_DATAin_flg)
  [VTPM_S2ID_raw32] -> LowerTirePressureCalibration/6(VTPM_S2ID_raw32)
  [VINP_TPMSResButt_flg] -> LowerTirePressureCalibration/9(VINP_TPMSResButt_flg)
  [VTPM_S3ID_raw32] -> LowerTirePressureCalibration/7(VTPM_S3ID_raw32)
  [VTPM_S4ID_raw32] -> LowerTirePressureCalibration/8(VTPM_S4ID_raw32)
  [VINP_TPMSStorge_flg] -> LowerTirePressureCalibration/11(VINP_TPMSStorge_flg)
  [VINP_ChkStorge_flg] -> LowerTirePressureCalibration/12(VINP_ChkStorge_flg)
  [VTPM_IDLOCK_flg] -> LowerTirePressureCalibration/10(VTPM_IDLOCK_flg)
  [VTPM_S1timeout_flg] -> LowerTirePressureCalibration/13(VTPM_S1timeout_flg)
  [VTPM_S2timeout_flg] -> LowerTirePressureCalibration/14(VTPM_S2timeout_flg)
  [VTPM_S3timeout_flg] -> LowerTirePressureCalibration/15(VTPM_S4timeout_flg)
  [VTPM_S4timeout_flg] -> LowerTirePressureCalibration/16(VTPM_S3timeout_flg)
  VINP_TPMSCaliButt_flg/1 -> LowerTirePressureCalibration/17(VINP_TPMSCaliButt_flg)
  VINP_FlashLFWheelPSW_raw8/1 -> LowerTirePressureCalibration/18(VINP_FlashLFWheelPSW_raw8)
  VINP_FlashRFWheelPSW_raw8/1 -> LowerTirePressureCalibration/19(VINP_FlashRFWheelPSW_raw8)
  VINP_FlashLRWheelPSW_raw8/1 -> LowerTirePressureCalibration/20(VINP_FlashLRWheelPSW_raw8)
  VINP_FlashRRWheelPSW_raw8/1 -> LowerTirePressureCalibration/21(VINP_FlashRRWheelPSW_raw8)
  VINP_FlashLFPindi_enum/1 -> LowerTirePressureCalibration/22(VINP_FlashLFPindi_enum)
  VINP_FlashRFPindi_enum/1 -> LowerTirePressureCalibration/23(VINP_FlashRFPindi_enum)
  VINP_FlashLRPindi_enum/1 -> LowerTirePressureCalibration/24(VINP_FlashLRPindi_enum)
  VINP_FlashRRPindi_enum/1 -> LowerTirePressureCalibration/25(VINP_FlashRRPindi_enum)
  [VTPM_IDLOCK_flg] -> VTPM_IDLOCK_flg/1
  [VINP_DATAin_flg] -> AutoLocation/3(VINP_DATAin_flg)
  [VINP_IDin_raw32] -> AutoLocation/2(VINP_IDin_raw32)
  [VINP_TPMSResButt_flg] -> AutoLocation/1(VINP_TPMSResButt_flg)
  VINP_FAT_flg/1 -> AutoLocation/4(VINP_FAT_flg)
  VPMM_PowerSta_enum/1 -> AutoLocation/5(VPMM_PowerSta_enum)
  VINP_LFPulseCount_cnt/1 -> AutoLocation/6(VINP_LFPulseCount_cnt)
  VINP_RFPulseCount_cnt/1 -> AutoLocation/7(VINP_RFPulseCount_cnt)
  VINP_LRPulseCount_cnt/1 -> AutoLocation/8(VINP_LRPulseCount_cnt)
  VINP_RRPulseCount_cnt/1 -> AutoLocation/9(VINP_RRPulseCount_cnt)
  VINP_LFPulseCountV_flg/1 -> AutoLocation/10(VINP_LFPulseCountV_flg)
  VINP_RFPulseCountV_flg/1 -> AutoLocation/11(VINP_RFPulseCountV_flg)
  VINP_LRPulseCountV_flg/1 -> AutoLocation/12(VINP_LRPulseCountV_flg)
  VINP_RRPulseCountV_flg/1 -> AutoLocation/13(VINP_RRPulseCountV_flg)
  VTPM_LFWhlRotDir_enum/1 -> AutoLocation/14(VTPM_LFWhlRotDir_enum)
  VTPM_RFWhlRotDir_enum/1 -> AutoLocation/15(VTPM_RFWhlRotDir_enum)
  VTPM_LRWhlRotDir_enum/1 -> AutoLocation/16(VTPM_LRWhlRotDir_enum)
  VTPM_RRWhlRotDir_enum/1 -> AutoLocation/17(VTPM_RRWhlRotDir_enum)
  [VINP_TPMSStorge_flg] -> AutoLocation/18(VINP_TPMSStorge_flg)
  [VINP_ChkStorge_flg] -> AutoLocation/23(VINP_ChkStorge_flg)
  VINP_LFID_raw/1 -> AutoLocation/19(VINP_LFID_raw)
  VINP_RFID_raw/1 -> AutoLocation/20(VINP_RFID_raw)
  VINP_LRID_raw/1 -> AutoLocation/21(VINP_LRID_raw)
  VINP_RRID_raw/1 -> AutoLocation/22(VINP_RRID_raw)
  VINP_ChkLFID_raw/1 -> AutoLocation/24(VINP_ChkLFID_raw)
  VINP_ChkRFID_raw/1 -> AutoLocation/25(VINP_ChkRFID_raw)
  VINP_ChkLRID_raw/1 -> AutoLocation/26(VINP_ChkLRID_raw)
  VINP_ChkRRID_raw/1 -> AutoLocation/27(VINP_ChkRRID_raw)
  VINP_VehSpeed_kph/1 -> AutoLocation/28(VINP_VehSpeed_kph)
  VINP_FlashunlearnSfali_flg/1 -> AutoLocation/29(VINP_FlashunlearnSfali_flg)
  VINP_S1ID_raw/1 -> AutoLocation/30(VINP_S1ID_raw)
  VINP_S2ID_raw/1 -> AutoLocation/31(VINP_S2ID_raw)
  VINP_S3ID_raw/1 -> AutoLocation/32(VINP_S3ID_raw)
  VINP_S4ID_raw/1 -> AutoLocation/33(VINP_S4ID_raw)
  [VINP_Pin_raw8] -> AutoLocation/34(VINP_Pin_raw8)
  [VINP_Tin_raw8] -> AutoLocation/35(VINP_Tin_raw8)
  VINP_TPMSTrigger_flg/1 -> AutoLocation/36(VINP_TPMSTrigger_flg)
  [VTPM_DiagLearn_flg] -> AutoLocation/37(VTPM_DiagLearn_flg)
  AutoLocation/1(VTPM_S1L_enum) -> [VTPM_S1L_enum], VTPM_S1L_enum/1
  AutoLocation/2(S1ID) -> [VTPM_S1ID_raw32]
  AutoLocation/3(VTPM_S2L_enum) -> [VTPM_S2L_enum], VTPM_S2L_enum/1
  AutoLocation/4(S2ID) -> [VTPM_S2ID_raw32]
  AutoLocation/5(VTPM_S3L_enum) -> [VTPM_S3L_enum], VTPM_S3L_enum/1
  AutoLocation/6(S3ID) -> [VTPM_S3ID_raw32]
  AutoLocation/8(S4ID) -> [VTPM_S4ID_raw32]
  AutoLocation/9(VTPM_LFS1_cnt) -> VTPM_LFS1_cnt/1
  AutoLocation/10(VTPM_RFS1_cnt) -> VTPM_RFS1_cnt/1
  AutoLocation/11(VTPM_RRS1_cnt) -> VTPM_RRS1_cnt/1
  AutoLocation/12(VTPM_LRS1_cnt) -> VTPM_LRS1_cnt/1
  AutoLocation/13(VTPM_LFS2_cnt) -> VTPM_LFS2_cnt/1
  AutoLocation/14(VTPM_RFS2_cnt) -> VTPM_RFS2_cnt/1
  AutoLocation/15(VTPM_RRS2_cnt) -> VTPM_RRS2_cnt/1
  AutoLocation/16(VTPM_LRS2_cnt) -> VTPM_LRS2_cnt/1
  AutoLocation/17(VTPM_LFS3_cnt) -> VTPM_LFS3_cnt/1
  AutoLocation/18(VTPM_RFS3_cnt) -> VTPM_RFS3_cnt/1
  AutoLocation/19(VTPM_RRS3_cnt) -> VTPM_RRS3_cnt/1
  AutoLocation/20(VTPM_LRS3_cnt) -> VTPM_LRS3_cnt/1
  AutoLocation/21(VTPM_LFS4_cnt) -> VTPM_LFS4_cnt/1
  AutoLocation/22(VTPM_RFS4_cnt) -> VTPM_RFS4_cnt/1
  AutoLocation/23(VTPM_RRS4_cnt) -> VTPM_RRS4_cnt/1
  AutoLocation/24(VTPM_LRS4_cnt) -> VTPM_LRS4_cnt/1
  AutoLocation/25(VTPM_IDLOCK_flg) -> [VTPM_IDLOCK_flg]
  AutoLocation/26(VINP_FATAND_flg) -> VTPM_FATAND_flg/1
  AutoLocation/27(VTPM_ALLFin_flg) -> VTPM_ALFin_flg/1
  AutoLocation/28(VTPM_S1WheelDebugALTU_pct) -> VTPM_S1WheelDebugALTU_pct/1
  AutoLocation/29(VTPM_S2WheelDebugALTU_pct) -> VTPM_S2WheelDebugALTU_pct/1
  AutoLocation/30(VTPM_S3WheelDebugALTU_pct) -> VTPM_S3WheelDebugALTU_pct/1
  AutoLocation/31(VTPM_S4WheelDebugALTU_pct) -> VTPM_S4WheelDebugALTU_pct/1
  AutoLocation/32(VTPM_ID1messageALTU_raw8) -> VTPM_ID1messageALTU_raw8/1
  AutoLocation/33(VTPM_ID2messageALTU_raw8) -> VTPM_ID2messageALTU_raw8/1
  AutoLocation/34(VTPM_ID3messageALTU_raw8) -> VTPM_ID3messageALTU_raw8/1
  AutoLocation/35(VTPM_ID4messageALTU_raw8) -> VTPM_ID4messageALTU_raw8/1
  AutoLocation/36(VTPM_SetIDLoc_flg) -> VTPM_SetIDLoc_flg/1
  AutoLocation/37(VTPM_Chkfin_flg) -> VTPM_Chkfin_flg/1
  AutoLocation/38(VTPM_unlearnSfali_flg) -> VTPM_unlearnSfali_flg/1
  AutoLocation/39(VTPM_unlearnSfailvalid_enum) -> VTPM_unlearnSfailvalid_enum/1
  AutoLocation/40(VTPM_FlashS1ID_raw) -> VTPM_FlashS1ID_raw/1
  AutoLocation/41(VTPM_FlashS2ID_raw) -> VTPM_FlashS2ID_raw/1
  AutoLocation/42(VTPM_FlashS3ID_raw) -> VTPM_FlashS3ID_raw/1
  AutoLocation/43(VTPM_FlashS4ID_raw) -> VTPM_FlashS4ID_raw/1
  AutoLocation/44(VTPM_FlashIDvalid_enum) -> VTPM_FlashIDvalid_enum/1
  AutoLocation/45(VTPM_S1timeout_flg) -> [VTPM_S1timeout_flg]
  AutoLocation/46(VTPM_S2timeout_flg) -> [VTPM_S2timeout_flg]
  AutoLocation/47(VTPM_S3timeout_flg) -> [VTPM_S3timeout_flg]
  AutoLocation/48(VTPM_S4timeout_flg) -> [VTPM_S4timeout_flg]
  AutoLocation/49(VTPM_unlockpopup_flg) -> VTPM_unlockpopup_flg/1
  AutoLocation/57(VTPM_ManualID4Temp_C) -> [VTPM_ManualID4Temp_C], VTPM_ManualID4Temp_C/1
  AutoLocation/50(VTPM_ManualID1pressure_raw) -> [VTPM_ManualID1pressure_raw], VTPM_ManualID1pressure_raw/1
  AutoLocation/59(VTPM_WritingCnt_enum) -> VTPM_WritingCnt_enum/1
  AutoLocation/54(VTPM_ManualID1Temp_C) -> [VTPM_ManualID1Temp_C], VTPM_ManualID1Temp_C/1
  AutoLocation/56(VTPM_ManualID3Temp_C) -> [VTPM_ManualID3Temp_C], VTPM_ManualID3Temp_C/1
  AutoLocation/53(VTPM_ManualID4pressure_raw) -> [VTPM_ManualID4pressure_raw], VTPM_ManualID4pressure_raw/1
  AutoLocation/55(VTPM_ManualID2Temp_C) -> [VTPM_ManualID2Temp_C], VTPM_ManualID2Temp_C/1
  AutoLocation/52(VTPM_ManualID3pressure_raw) -> [VTPM_ManualID3pressure_raw], VTPM_ManualID3pressure_raw/1
  AutoLocation/58(VTPM_TPMSmanualDone_flg) -> VTPM_TPMSmanualDone_flg/1, [VTPM_TPMSmanualDone_flg]
  AutoLocation/51(VTPM_ManualID2pressure_raw) -> [VTPM_ManualID2pressure_raw], VTPM_ManualID2pressure_raw/1
  AutoLocation/60(VTPM_TPMSTLCmd_flg) -> VTPM_TPMSTLCmd_flg/1
  AutoLocation/61(VTPM_LProgress_enum) -> VTPM_LProgress_enum/1
  [VTPM_TPMSmanualDone_flg] -> LowerTirePressureCalibration/26(VTPM_TPMSmanualDone_flg)
  [VTPM_ManualID1pressure_raw] -> LowerTirePressureCalibration/27(VTPM_ManualID1pressure_raw)
  [VTPM_ManualID2pressure_raw] -> LowerTirePressureCalibration/28(VTPM_ManualID2pressure_raw)
  [VTPM_ManualID3pressure_raw] -> LowerTirePressureCalibration/29(VTPM_ManualID3pressure_raw)
  [VTPM_ManualID4pressure_raw] -> LowerTirePressureCalibration/30(VTPM_ManualID4pressure_raw)
  [VTPM_ManualID1Temp_C] -> LowerTirePressureCalibration/31(VTPM_ManualID1Temp_C)
  [VTPM_ManualID2Temp_C] -> LowerTirePressureCalibration/32(VTPM_ManualID2Temp_C)
  [VTPM_ManualID3Temp_C] -> LowerTirePressureCalibration/33(VTPM_ManualID3Temp_C)
  [VTPM_ManualID4Temp_C] -> LowerTirePressureCalibration/34(VTPM_ManualID4Temp_C)
  [VTPM_DiagLearn_flg] -> LowerTirePressureCalibration/35(VTPM_DiagLearn_flg)
  VTPM_DiagLearn_flg/1 -> [VTPM_DiagLearn_flg]
  AutoLocation/7(VTPM_S4L_enum) -> [VTPM_S4L_enum], VTPM_S4L_enum/1
  [VTPM_S1L_enum] -> LowerTirePressureCalibration/36(VTPM_S1L_enum)
  [VTPM_S2L_enum] -> LowerTirePressureCalibration/37(VTPM_S2L_enum)
  [VTPM_S3L_enum] -> LowerTirePressureCalibration/38(VTPM_S3L_enum)
  [VTPM_S4L_enum] -> LowerTirePressureCalibration/39(VTPM_S4L_enum)
  LowerTirePressureCalibration/1(VTPM_LFWheelPSW_raw8) -> VTPM_LFWheelPSW_raw8/1
  LowerTirePressureCalibration/2(VTPM_RFWheelPSW_raw8) -> VTPM_RFWheelPSW_raw8/1
  LowerTirePressureCalibration/3(VTPM_LRWheelPSW_raw8) -> VTPM_LRWheelPSW_raw8/1
  LowerTirePressureCalibration/4(VTPM_RRWheelPSW_raw8) -> VTPM_RRWheelPSW_raw8/1
  LowerTirePressureCalibration/5(VTPM_LFLowPind_enum) -> VTPM_LFLowPind_enum/1
  LowerTirePressureCalibration/6(VTPM_RFLowPind_enum) -> VTPM_RFLowPind_enum/1
  LowerTirePressureCalibration/7(VTPM_LRLowPind_enum) -> VTPM_LRLowPind_enum/1
  LowerTirePressureCalibration/8(VTPM_RRLowPind_enum) -> VTPM_RRLowPind_enum/1
  LowerTirePressureCalibration/12(VTPM_ManualRRP20_raw8) -> VTPM_ManualRRP20_raw8/1
  LowerTirePressureCalibration/11(VTPM_ManualLRP20_raw8) -> VTPM_ManualLRP20_raw8/1
  LowerTirePressureCalibration/10(VTPM_ManualRFP20_raw8) -> VTPM_ManualRFP20_raw8/1
  LowerTirePressureCalibration/9(VTPM_ManualLFP20_raw8) -> VTPM_ManualLFP20_raw8/1
